simulink model "VIPLExit557StEnCtrl"  (R2018b)
settings: Solver=FixedStepDiscrete  StartTime=0.0  StopTime=10.0  FixedStep=0.01  RelTol=1e-3
undefined symbols (not defined in the file or in its folder): data, KeSMSw4SSecRwLtStLgrstOtwdInwdClosePos1_Val, KeSMSw4SSecRwLtStLgrstUpwdDnwdClosePos1_Val, KeSMSw4SSecRwLtStLgrstUpwdDnwdClosePos2_Val, KeSMSw4SSecRwLtStLgrstUpwdDnwdOpenPos1_Val, SecRwLtStBkReclnEn_Clear, SecRwLtStBkReclnEn_Set, SecRwLtStFwdBkwdEn_Clear, SecRwLtStFwdBkwdEn_Set, SecRwLtStLgrstInwdOtwdEn_Clear, SecRwLtStLgrstInwdOtwdEn_Set, SecRwLtStLgrstUpwdDnwdEn_Clear, SecRwLtStLgrstUpwdDnwdEn_Set, ThdRwLtStBkReclnEn_Clear, ThdRwLtStBkReclnEn_Set, ThdRwLtStFwdBkwdEn_Clear, ThdRwLtStFwdBkwdEn_Set, ZeroLEn_Clear, ZeroLEn_Set
libraries: simulink x1
settings Model: Creator=sn2xws  LastModifiedBy=sn2xws
settings Model: ModifiedHistory=|
  | 2024.7.2 V3.0.0 557模式流程V1.9
  | 2024.8.21 V3.0.1 增加FitstTrig参数
  | 2024.9.18 V3.0.2 三排占座应不动三排，第三阶段遗漏三排靠背动作
  | 2024.10.8 V3.0.3方向比较类型设置错误
settings DataIOCC: SaveFormat=StructureWithTime
settings OptimizationCC: DefaultParameterBehavior=Inlined  EnhancedBackFolding=on  PassReuseOutputArgsAs=Individual arguments  ZeroExternalMemoryAtStartup=off  ZeroInternalMemoryAtStartup=off  OptimizeBlockOrder=speed  DifferentSizesBufferReuse=on  OptimizationCustomize=off
settings DebuggingCC: ParameterTunabilityLossMsg=error
settings SFSimCC: MATLABDynamicMemAlloc=off
settings RTWCC: SystemTargetFile=autosar.tlc  GenCodeOnly=on  TemplateMakefile=ert_default_tmf  Description=AUTOSAR  GenerateReport=on  IncludeHyperlinkInReport=on  LaunchReport=on  GenerateTraceInfo=on  GenerateTraceReport=on  GenerateTraceReportSl=on  GenerateTraceReportSf=on  GenerateTraceReportEml=on
settings CodeAppCC: ForceParamTrailComments=on  IgnoreCustomStorageClasses=off  OperatorAnnotations=on  SimulinkDataObjDesc=on  SFDataObjDesc=on  InsertBlockDesc=on
settings STFCustomTargetCC: TargetLangStandard=C99 (ISO)  MultiwordLength=256  ParMdlRefBuildCompliant=on  CompOptLevelCompliant=on  IncludeMdlTerminateFcn=off  CombineOutputUpdateFcns=on  SuppressErrorStatus=on  ERTCustomFileBanners=on  SupportNonFinite=off  SupportComplex=off  SupportContinuousTime=off  SupportNonInlinedSFcns=off  RemoveResetFunc=on  MATLABClassNameForMDSCustomization=Simulink.SoftwareTarget.ERTCustomization  AutosarCompliant=on  UseToolchainInfoCompliant=on  LookupTableObjectStructAxisOrder=2,1,3,4,...  LUTObjectStructOrderEvenSpacing=Size,Table,Breakpoints  SystemTargetFile=autosar.tlc
settings ERTTargetCC: TargetLangStandard=C99 (ISO)  ConcurrentExecutionCompliant=off  IncludeMdlTerminateFcn=off  SuppressErrorStatus=on  SupportNonFinite=off  SupportComplex=off  ModelStepFunctionPrototypeControlCompliant=off  CPPClassGenCompliant=off  AutosarCompliant=on  LookupTableObjectStructAxisOrder=2,1,3,4,...  LUTObjectStructOrderEvenSpacing=Size,Table,Breakpoints  InlinedParameterPlacement=NonHierarchical  ERTCustomFileTemplate=example_file_process.tlc  ERTFilePackagingFormat=Compact

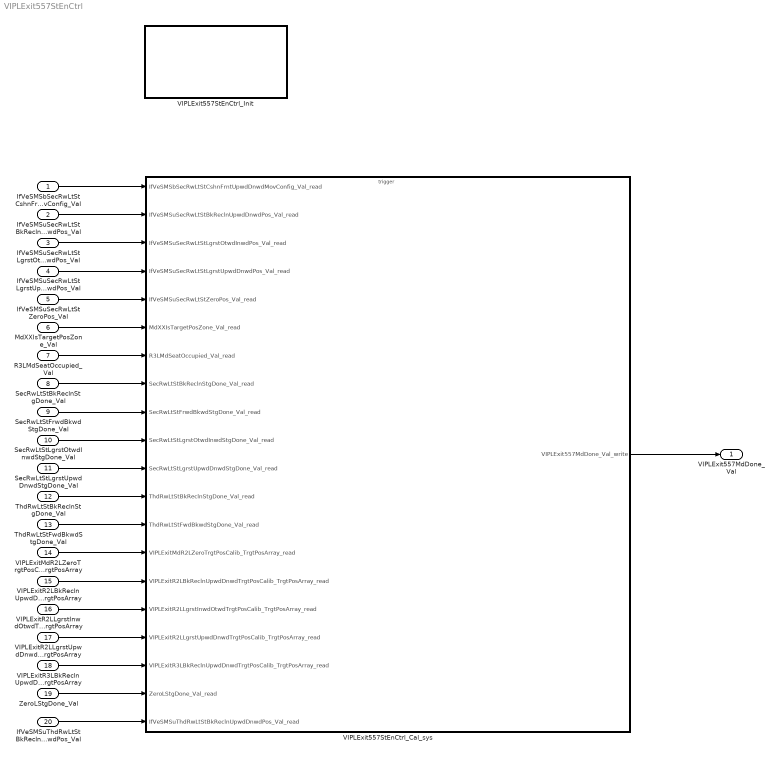
== system VIPLExit557StEnCtrl ==
  IfVeSMSbSecRwLtStCshnFrntUpwdDnwdMovConfig_Val : Inport  OutDataTypeStr=boolean  PortDimensions=1
  IfVeSMSuSecRwLtStBkReclnUpwdDnwdPos_Val : Inport  Port=2  OutDataTypeStr=uint16  PortDimensions=1
  IfVeSMSuSecRwLtStLgrstOtwdInwdPos_Val : Inport  Port=3  OutDataTypeStr=uint16  PortDimensions=1
  IfVeSMSuSecRwLtStLgrstUpwdDnwdPos_Val : Inport  Port=4  OutDataTypeStr=uint16  PortDimensions=1
  IfVeSMSuSecRwLtStZeroPos_Val : Inport  Port=5  OutDataTypeStr=uint16  PortDimensions=1
  MdXXIsTargetPosZone_Val : Inport  Port=6  OutDataTypeStr=uint32  PortDimensions=1
  R3LMdSeatOccupied_Val : Inport  Port=7  OutDataTypeStr=boolean  PortDimensions=1
  SecRwLtStBkReclnStgDone_Val : Inport  Port=8  OutDataTypeStr=boolean  PortDimensions=1
  SecRwLtStFrwdBkwdStgDone_Val : Inport  Port=9  OutDataTypeStr=boolean  PortDimensions=1
  SecRwLtStLgrstOtwdInwdStgDone_Val : Inport  Port=10  OutDataTypeStr=boolean  PortDimensions=1
  SecRwLtStLgrstUpwdDnwdStgDone_Val : Inport  Port=11  OutDataTypeStr=boolean  PortDimensions=1
  ThdRwLtStBkReclnStgDone_Val : Inport  Port=12  OutDataTypeStr=boolean  PortDimensions=1
  ThdRwLtStFwdBkwdStgDone_Val : Inport  Port=13  OutDataTypeStr=boolean  PortDimensions=1
  VIPLExitMdR2LZeroTrgtPosCalib_TrgtPosArray : Inport  Description=|  Port=14  OutDataTypeStr=uint16  PortDimensions=3
      | 0:Pos
      | 1:Max
      | 2:Min
  VIPLExitR2LBkReclnUpwdDnwdTrgtPosCalib_TrgtPosArray : Inport  Description=|  Port=15  OutDataTypeStr=uint16  PortDimensions=3
      | 0:Pos
      | 1:Max
      | 2:Min
  VIPLExitR2LLgrstInwdOtwdTrgtPosCalib_TrgtPosArray : Inport  Description=|  Port=16  OutDataTypeStr=uint16  PortDimensions=3
      | 0:Pos
      | 1:Max
      | 2:Min
  VIPLExitR2LLgrstUpwdDnwdTrgtPosCalib_TrgtPosArray : Inport  Description=|  Port=17  OutDataTypeStr=uint16  PortDimensions=3
      | 0:Pos
      | 1:Max
      | 2:Min
  VIPLExitR3LBkReclnUpwdDnwdTrgtPosCalib_TrgtPosArray : Inport  Description=|  Port=18  OutDataTypeStr=uint16  PortDimensions=3
      | 0:Pos
      | 1:Max
      | 2:Min
  ZeroLStgDone_Val : Inport  Port=19  OutDataTypeStr=boolean  PortDimensions=1
  IfVeSMSuThdRwLtStBkReclnUpwdDnwdPos_Val : Inport  Port=20  OutDataTypeStr=uint16  PortDimensions=1
  VIPLExit557StEnCtrl_Cal_sys : Subsystem
  VIPLExit557StEnCtrl_Init : Subsystem
  VIPLExit557MdDone_Val : Outport  OutDataTypeStr=uint8  PortDimensions=1
  wires:
  IfVeSMSbSecRwLtStCshnFrntUpwdDnwdMovConfig_Val/1 -> VIPLExit557StEnCtrl_Cal_sys/1(IfVeSMSbSecRwLtStCshnFrntUpwdDnwdMovConfig_Val_read)
  IfVeSMSuSecRwLtStBkReclnUpwdDnwdPos_Val/1 -> VIPLExit557StEnCtrl_Cal_sys/2(IfVeSMSuSecRwLtStBkReclnUpwdDnwdPos_Val_read)
  IfVeSMSuSecRwLtStLgrstOtwdInwdPos_Val/1 -> VIPLExit557StEnCtrl_Cal_sys/3(IfVeSMSuSecRwLtStLgrstOtwdInwdPos_Val_read)
  IfVeSMSuSecRwLtStLgrstUpwdDnwdPos_Val/1 -> VIPLExit557StEnCtrl_Cal_sys/4(IfVeSMSuSecRwLtStLgrstUpwdDnwdPos_Val_read)
  IfVeSMSuSecRwLtStZeroPos_Val/1 -> VIPLExit557StEnCtrl_Cal_sys/5(IfVeSMSuSecRwLtStZeroPos_Val_read)
  MdXXIsTargetPosZone_Val/1 -> VIPLExit557StEnCtrl_Cal_sys/6(MdXXIsTargetPosZone_Val_read)
  R3LMdSeatOccupied_Val/1 -> VIPLExit557StEnCtrl_Cal_sys/7(R3LMdSeatOccupied_Val_read)
  SecRwLtStBkReclnStgDone_Val/1 -> VIPLExit557StEnCtrl_Cal_sys/8(SecRwLtStBkReclnStgDone_Val_read)
  SecRwLtStFrwdBkwdStgDone_Val/1 -> VIPLExit557StEnCtrl_Cal_sys/9(SecRwLtStFrwdBkwdStgDone_Val_read)
  SecRwLtStLgrstOtwdInwdStgDone_Val/1 -> VIPLExit557StEnCtrl_Cal_sys/10(SecRwLtStLgrstOtwdInwdStgDone_Val_read)
  SecRwLtStLgrstUpwdDnwdStgDone_Val/1 -> VIPLExit557StEnCtrl_Cal_sys/11(SecRwLtStLgrstUpwdDnwdStgDone_Val_read)
  ThdRwLtStBkReclnStgDone_Val/1 -> VIPLExit557StEnCtrl_Cal_sys/12(ThdRwLtStBkReclnStgDone_Val_read)
  ThdRwLtStFwdBkwdStgDone_Val/1 -> VIPLExit557StEnCtrl_Cal_sys/13(ThdRwLtStFwdBkwdStgDone_Val_read)
  VIPLExitMdR2LZeroTrgtPosCalib_TrgtPosArray/1 -> VIPLExit557StEnCtrl_Cal_sys/14(VIPLExitMdR2LZeroTrgtPosCalib_TrgtPosArray_read)
  VIPLExitR2LBkReclnUpwdDnwdTrgtPosCalib_TrgtPosArray/1 -> VIPLExit557StEnCtrl_Cal_sys/15(VIPLExitR2LBkReclnUpwdDnwdTrgtPosCalib_TrgtPosArray_read)
  VIPLExitR2LLgrstInwdOtwdTrgtPosCalib_TrgtPosArray/1 -> VIPLExit557StEnCtrl_Cal_sys/16(VIPLExitR2LLgrstInwdOtwdTrgtPosCalib_TrgtPosArray_read)
  VIPLExitR2LLgrstUpwdDnwdTrgtPosCalib_TrgtPosArray/1 -> VIPLExit557StEnCtrl_Cal_sys/17(VIPLExitR2LLgrstUpwdDnwdTrgtPosCalib_TrgtPosArray_read)
  VIPLExitR3LBkReclnUpwdDnwdTrgtPosCalib_TrgtPosArray/1 -> VIPLExit557StEnCtrl_Cal_sys/18(VIPLExitR3LBkReclnUpwdDnwdTrgtPosCalib_TrgtPosArray_read)
  ZeroLStgDone_Val/1 -> VIPLExit557StEnCtrl_Cal_sys/19(ZeroLStgDone_Val_read)
  VIPLExit557StEnCtrl_Cal_sys/1(VIPLExit557MdDone_Val_write) -> VIPLExit557MdDone_Val/1
  IfVeSMSuThdRwLtStBkReclnUpwdDnwdPos_Val/1 -> VIPLExit557StEnCtrl_Cal_sys/20(IfVeSMSuThdRwLtStBkReclnUpwdDnwdPos_Val_read)

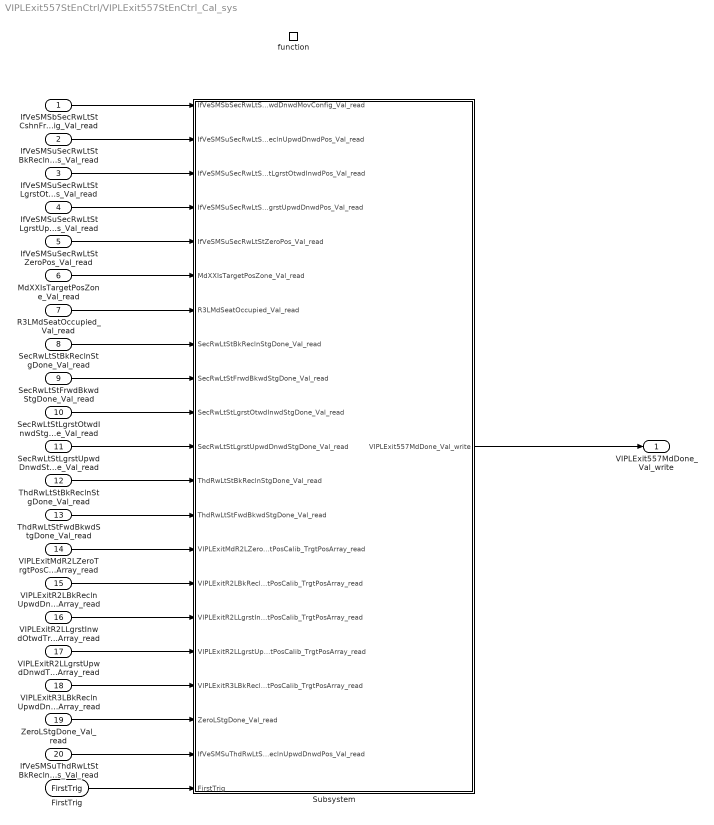
== system VIPLExit557StEnCtrl/VIPLExit557StEnCtrl_Cal_sys ==
  IfVeSMSbSecRwLtStCshnFrntUpwdDnwdMovConfig_Val_read : Inport
  IfVeSMSuSecRwLtStBkReclnUpwdDnwdPos_Val_read : Inport  Port=2
  IfVeSMSuSecRwLtStLgrstOtwdInwdPos_Val_read : Inport  Port=3
  IfVeSMSuSecRwLtStLgrstUpwdDnwdPos_Val_read : Inport  Port=4
  IfVeSMSuSecRwLtStZeroPos_Val_read : Inport  Port=5
  MdXXIsTargetPosZone_Val_read : Inport  Port=6
  R3LMdSeatOccupied_Val_read : Inport  Port=7
  SecRwLtStBkReclnStgDone_Val_read : Inport  Port=8
  SecRwLtStFrwdBkwdStgDone_Val_read : Inport  Port=9
  SecRwLtStLgrstOtwdInwdStgDone_Val_read : Inport  Port=10
  SecRwLtStLgrstUpwdDnwdStgDone_Val_read : Inport  Port=11
  ThdRwLtStBkReclnStgDone_Val_read : Inport  Port=12
  ThdRwLtStFwdBkwdStgDone_Val_read : Inport  Port=13
  VIPLExitMdR2LZeroTrgtPosCalib_TrgtPosArray_read : Inport  Port=14
  VIPLExitR2LBkReclnUpwdDnwdTrgtPosCalib_TrgtPosArray_read : Inport  Port=15
  VIPLExitR2LLgrstInwdOtwdTrgtPosCalib_TrgtPosArray_read : Inport  Port=16
  VIPLExitR2LLgrstUpwdDnwdTrgtPosCalib_TrgtPosArray_read : Inport  Port=17
  VIPLExitR3LBkReclnUpwdDnwdTrgtPosCalib_TrgtPosArray_read : Inport  Port=18
  ZeroLStgDone_Val_read : Inport  Port=19
  IfVeSMSuThdRwLtStBkReclnUpwdDnwdPos_Val_read : Inport  Port=20
  function : TriggerPort  TriggerType=function-call  IsSimulinkFunction=on  FunctionName=VIPLExit557StEnCtrl_Cal  VariantControl=(inherit)
  Subsystem : Subsystem
  FirstTrig : ArgIn  OutDataTypeStr=boolean  ArgumentName=FirstTrig
  VIPLExit557MdDone_Val_write : Outport
      settings: EnsureOutportIsVirtual=on
  wires:
  IfVeSMSbSecRwLtStCshnFrntUpwdDnwdMovConfig_Val_read/1 -> Subsystem/1(IfVeSMSbSecRwLtStCshnFrntUpwdDnwdMovConfig_Val_read)
  IfVeSMSuSecRwLtStBkReclnUpwdDnwdPos_Val_read/1 -> Subsystem/2(IfVeSMSuSecRwLtStBkReclnUpwdDnwdPos_Val_read)
  IfVeSMSuSecRwLtStLgrstOtwdInwdPos_Val_read/1 -> Subsystem/3(IfVeSMSuSecRwLtStLgrstOtwdInwdPos_Val_read)
  IfVeSMSuSecRwLtStLgrstUpwdDnwdPos_Val_read/1 -> Subsystem/4(IfVeSMSuSecRwLtStLgrstUpwdDnwdPos_Val_read)
  IfVeSMSuSecRwLtStZeroPos_Val_read/1 -> Subsystem/5(IfVeSMSuSecRwLtStZeroPos_Val_read)
  MdXXIsTargetPosZone_Val_read/1 -> Subsystem/6(MdXXIsTargetPosZone_Val_read)
  R3LMdSeatOccupied_Val_read/1 -> Subsystem/7(R3LMdSeatOccupied_Val_read)
  SecRwLtStBkReclnStgDone_Val_read/1 -> Subsystem/8(SecRwLtStBkReclnStgDone_Val_read)
  SecRwLtStFrwdBkwdStgDone_Val_read/1 -> Subsystem/9(SecRwLtStFrwdBkwdStgDone_Val_read)
  SecRwLtStLgrstOtwdInwdStgDone_Val_read/1 -> Subsystem/10(SecRwLtStLgrstOtwdInwdStgDone_Val_read)
  SecRwLtStLgrstUpwdDnwdStgDone_Val_read/1 -> Subsystem/11(SecRwLtStLgrstUpwdDnwdStgDone_Val_read)
  ThdRwLtStBkReclnStgDone_Val_read/1 -> Subsystem/12(ThdRwLtStBkReclnStgDone_Val_read)
  ThdRwLtStFwdBkwdStgDone_Val_read/1 -> Subsystem/13(ThdRwLtStFwdBkwdStgDone_Val_read)
  VIPLExitMdR2LZeroTrgtPosCalib_TrgtPosArray_read/1 -> Subsystem/14(VIPLExitMdR2LZeroTrgtPosCalib_TrgtPosArray_read)
  VIPLExitR2LBkReclnUpwdDnwdTrgtPosCalib_TrgtPosArray_read/1 -> Subsystem/15(VIPLExitR2LBkReclnUpwdDnwdTrgtPosCalib_TrgtPosArray_read)
  VIPLExitR2LLgrstInwdOtwdTrgtPosCalib_TrgtPosArray_read/1 -> Subsystem/16(VIPLExitR2LLgrstInwdOtwdTrgtPosCalib_TrgtPosArray_read)
  VIPLExitR2LLgrstUpwdDnwdTrgtPosCalib_TrgtPosArray_read/1 -> Subsystem/17(VIPLExitR2LLgrstUpwdDnwdTrgtPosCalib_TrgtPosArray_read)
  VIPLExitR3LBkReclnUpwdDnwdTrgtPosCalib_TrgtPosArray_read/1 -> Subsystem/18(VIPLExitR3LBkReclnUpwdDnwdTrgtPosCalib_TrgtPosArray_read)
  ZeroLStgDone_Val_read/1 -> Subsystem/19(ZeroLStgDone_Val_read)
  Subsystem/1(VIPLExit557MdDone_Val_write) -> VIPLExit557MdDone_Val_write/1
  IfVeSMSuThdRwLtStBkReclnUpwdDnwdPos_Val_read/1 -> Subsystem/20(IfVeSMSuThdRwLtStBkReclnUpwdDnwdPos_Val_read)
  FirstTrig/1 -> Subsystem/21(FirstTrig)

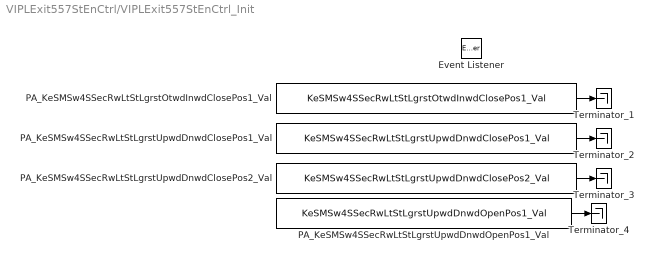
== system VIPLExit557StEnCtrl/VIPLExit557StEnCtrl_Init ==
  Event Listener : EventListener  EventName=reset
  PA_KeSMSw4SSecRwLtStLgrstOtwdInwdClosePos1_Val : Constant  Value=KeSMSw4SSecRwLtStLgrstOtwdInwdClosePos1_Val
  PA_KeSMSw4SSecRwLtStLgrstUpwdDnwdClosePos1_Val : Constant  Value=KeSMSw4SSecRwLtStLgrstUpwdDnwdClosePos1_Val
  PA_KeSMSw4SSecRwLtStLgrstUpwdDnwdClosePos2_Val : Constant  Value=KeSMSw4SSecRwLtStLgrstUpwdDnwdClosePos2_Val
  PA_KeSMSw4SSecRwLtStLgrstUpwdDnwdOpenPos1_Val : Constant  Value=KeSMSw4SSecRwLtStLgrstUpwdDnwdOpenPos1_Val
  Terminator_{1..4} (4 alike) : Terminator
  wires:
  PA_KeSMSw4SSecRwLtStLgrstOtwdInwdClosePos1_Val/1 -> Terminator_1/1
  PA_KeSMSw4SSecRwLtStLgrstUpwdDnwdClosePos1_Val/1 -> Terminator_2/1
  PA_KeSMSw4SSecRwLtStLgrstUpwdDnwdClosePos2_Val/1 -> Terminator_3/1
  PA_KeSMSw4SSecRwLtStLgrstUpwdDnwdOpenPos1_Val/1 -> Terminator_4/1

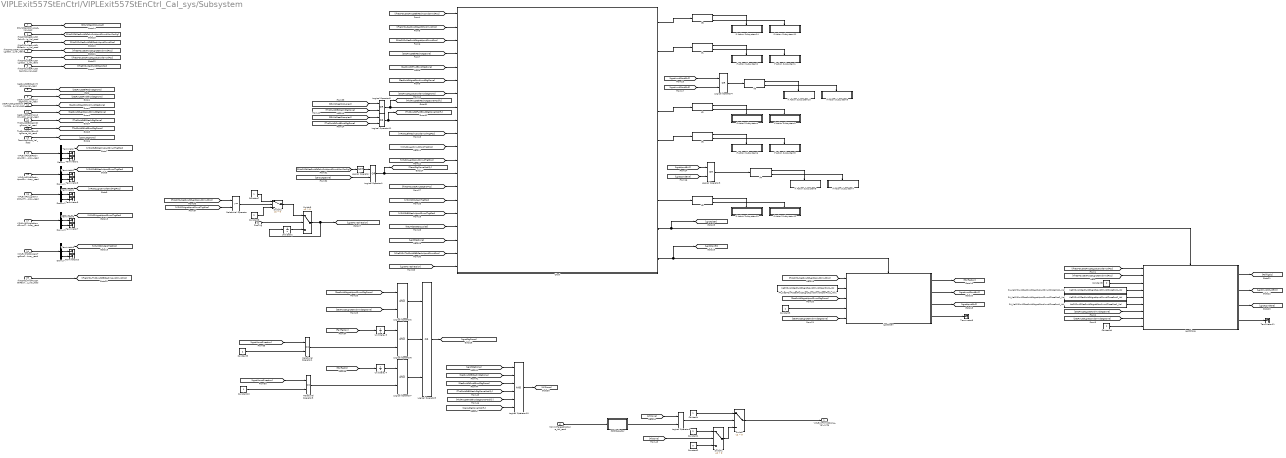
== system VIPLExit557StEnCtrl/VIPLExit557StEnCtrl_Cal_sys/Subsystem ==
  IfVeSMSbSecRwLtStCshnFrntUpwdDnwdMovConfig_Val_read : Inport
  IfVeSMSuSecRwLtStBkReclnUpwdDnwdPos_Val_read : Inport  Port=2
  IfVeSMSuSecRwLtStLgrstOtwdInwdPos_Val_read : Inport  Port=3
  IfVeSMSuSecRwLtStLgrstUpwdDnwdPos_Val_read : Inport  Port=4
  IfVeSMSuSecRwLtStZeroPos_Val_read : Inport  Port=5
  MdXXIsTargetPosZone_Val_read : Inport  Port=6
  R3LMdSeatOccupied_Val_read : Inport  Port=7
  SecRwLtStBkReclnStgDone_Val_read : Inport  Port=8
  SecRwLtStFrwdBkwdStgDone_Val_read : Inport  Port=9
  SecRwLtStLgrstOtwdInwdStgDone_Val_read : Inport  Port=10
  SecRwLtStLgrstUpwdDnwdStgDone_Val_read : Inport  Port=11
  ThdRwLtStBkReclnStgDone_Val_read : Inport  Port=12
  ThdRwLtStFwdBkwdStgDone_Val_read : Inport  Port=13
  VIPLExitMdR2LZeroTrgtPosCalib_TrgtPosArray_read : Inport  Port=14
  VIPLExitR2LBkReclnUpwdDnwdTrgtPosCalib_TrgtPosArray_read : Inport  Port=15
  VIPLExitR2LLgrstInwdOtwdTrgtPosCalib_TrgtPosArray_read : Inport  Port=16
  VIPLExitR2LLgrstUpwdDnwdTrgtPosCalib_TrgtPosArray_read : Inport  Port=17
  VIPLExitR3LBkReclnUpwdDnwdTrgtPosCalib_TrgtPosArray_read : Inport  Port=18
  ZeroLStgDone_Val_read : Inport  Port=19
  IfVeSMSuThdRwLtStBkReclnUpwdDnwdPos_Val_read : Inport  Port=20
  FirstTrig : Inport  Port=21
  32BitSelector : Subsystem  mask(32 Bit Selector){BitNum=26}
      mask prompts: BitNum "Select Bit Number"
      mask help: Allows selection of a particular bit (0-31) out of a packed word up to 32 bits long. Output will be true if the bit number selected via the mask parameter is equal to one.
      mask TypeOptions BitNum: 0 | 1 | 2 | 3 | 4 | 5 | 6 | 7 | 8 | 9 | 10 | 11 | 12 | 13 | 14 | 15 | 16 | 17 | 18 | 19 | 20 | 21 | 22 | 23 | 24 | 25 | 26 | 27 | 28 | 29 | 30 | 31
      mask Display:
      | text(0.5, 0.8,'BIT','horizontalAlignment','center')
      | text(0.5, 0.5,'SELECTOR','horizontalAlignment','center')
      | text(0.5, 0.2,['-- Bit ',char(get_param(gcb,'BitNum')),' --'],'horizontalAlignment','center')
  Chart : Stateflow chart  TreatAsAtomicUnit=on
  Constant : Constant  OutDataTypeStr=uint8
  Constant1 : Constant  Value=2  OutDataTypeStr=uint8
  Constant10 : Constant  OutDataTypeStr=uint8
  Constant2 : Constant  Value=0  OutDataTypeStr=uint8
  Constant3 : Constant  OutDataTypeStr=boolean
  Constant4 : Constant  OutDataTypeStr=boolean
  Constant5 : Constant  Value=0  OutDataTypeStr=uint16
  Constant7 : Constant  OutDataTypeStr=uint8
  Constant8 : Constant  Value=2  OutDataTypeStr=uint8
  Constant9 : Constant  Value=2  OutDataTypeStr=uint8
  Demux{,1..4} (5 alike) : Demux  Outputs=3
  If Action Subsystem1 : Subsystem  TreatAsAtomicUnit=on
  If Action Subsystem10 : Subsystem  TreatAsAtomicUnit=on
  If Action Subsystem11 : Subsystem  TreatAsAtomicUnit=on
  If Action Subsystem12 : Subsystem  TreatAsAtomicUnit=on
  If Action Subsystem13 : Subsystem  TreatAsAtomicUnit=on
  If Action Subsystem14 : Subsystem  TreatAsAtomicUnit=on
  If Action Subsystem2 : Subsystem  TreatAsAtomicUnit=on
  If Action Subsystem3 : Subsystem  TreatAsAtomicUnit=on
  If Action Subsystem4 : Subsystem  TreatAsAtomicUnit=on
  If Action Subsystem5 : Subsystem  TreatAsAtomicUnit=on
  If Action Subsystem6 : Subsystem  TreatAsAtomicUnit=on
  If Action Subsystem7 : Subsystem  TreatAsAtomicUnit=on
  If Action Subsystem8 : Subsystem  TreatAsAtomicUnit=on
  If Action Subsystem9 : Subsystem  TreatAsAtomicUnit=on
  If{1..6,8} (7 alike) : If  IfExpression=u1
  LgrstClose : Subsystem
  LgrstOpen : Subsystem
  Logical Operator : Logic  Operator=NOT  AllPortsSameDT=off  OutDataTypeStr=boolean
  Logical Operator{1,3..4,8,11} (5 alike) : Logic  Operator=OR  AllPortsSameDT=off  OutDataTypeStr=boolean
  Logical Operator10 : Logic  Inputs=6  AllPortsSameDT=off  OutDataTypeStr=boolean
  Logical Operator{2,6..7,9} (4 alike) : Logic  AllPortsSameDT=off  OutDataTypeStr=boolean
  Logical Operator5 : Logic  Operator=OR  Inputs=3  AllPortsSameDT=off  OutDataTypeStr=boolean
  PA_KeSMSw4SSecRwLtStLgrstOtwdInwdClosePos1_Val : Constant  Value=KeSMSw4SSecRwLtStLgrstOtwdInwdClosePos1_Val
  PA_KeSMSw4SSecRwLtStLgrstUpwdDnwdClosePos1_Val : Constant  Value=KeSMSw4SSecRwLtStLgrstUpwdDnwdClosePos1_Val
  PA_KeSMSw4SSecRwLtStLgrstUpwdDnwdClosePos2_Val : Constant  Value=KeSMSw4SSecRwLtStLgrstUpwdDnwdClosePos2_Val
  PA_KeSMSw4SSecRwLtStLgrstUpwdDnwdOpenPos1_Val1 : Constant  Value=KeSMSw4SSecRwLtStLgrstUpwdDnwdOpenPos1_Val
  Relational Operator : RelationalOperator  OutDataTypeStr=boolean  RndMeth=Simplest
  Relational Operator1 : RelationalOperator  Operator===  OutDataTypeStr=boolean  RndMeth=Simplest
  Relational Operator3 : RelationalOperator  Operator===  OutDataTypeStr=boolean  RndMeth=Simplest
  Switch{,1..2,5} (4 alike) : Switch  Criteria=u2 > Threshold
  Terminator{,1..11} (12 alike) : Terminator
  Unit Delay : UnitDelay  SampleTime=-1
  Unit Delay3 : UnitDelay  SampleTime=-1
  Unit Delay4 : UnitDelay  SampleTime=-1
  VIPLExit557MdDone_Val_write : Outport
      settings: EnsureOutportIsVirtual=on
  wires:
  Switch/1 -> VIPLExit557MdDone_Val_write/1
  Constant1/1 -> Switch1/1
  Constant/1 -> Switch/1
  Constant2/1 -> Switch1/3
  32BitSelector/1(y) -> Logical Operator9/2
  Switch1/1 -> Switch/3
  MdXXIsTargetPosZone_Val_read/1 -> 32BitSelector/1(x)
  [AllDone] -> Logical Operator9/1
  [AllDone] -> Switch1/2
  Logical Operator9/1 -> Switch/2
  ZeroLStgDone_Val_read/1 -> [ZeroLStgDone]
  IfVeSMSuSecRwLtStBkReclnUpwdDnwdPos_Val_read/1 -> [IfVeSMSuSecRwLtStBkReclnUpwdDnwdPos]
  SecRwLtStLgrstUpwdDnwdStgDone_Val_read/1 -> [SecRwLtStLgrstUpwdDnwdStgDone]
  IfVeSMSuSecRwLtStLgrstUpwdDnwdPos_Val_read/1 -> [IfVeSMSuSecRwLtStLgrstUpwdDnwdPos]
  SecRwLtStFrwdBkwdStgDone_Val_read/1 -> [SecRwLtStFrwdBkwdStgDone]
  IfVeSMSuSecRwLtStLgrstOtwdInwdPos_Val_read/1 -> [IfVeSMSuSecRwLtStLgrstOtwdInwdPos]
  SecRwLtStLgrstOtwdInwdStgDone_Val_read/1 -> [SecRwLtStLgrstOtwdInwdStgDone]
  ThdRwLtStBkReclnStgDone_Val_read/1 -> [ThdRwLtStBkReclnStgDone]
  ThdRwLtStFwdBkwdStgDone_Val_read/1 -> [ThdRwLtStFwdBkwdStgDone]
  SecRwLtStBkReclnStgDone_Val_read/1 -> [SecRwLtStBkReclnStgDone]
  IfVeSMSuSecRwLtStZeroPos_Val_read/1 -> [IfVeSMSuSecRwLtStZeroPos]
  Demux4/3 -> Terminator10/1
  VIPLExitR3LBkReclnUpwdDnwdTrgtPosCalib_TrgtPosArray_read/1 -> Demux/1
  Demux4/2 -> Terminator9/1
  VIPLExitMdR2LZeroTrgtPosCalib_TrgtPosArray_read/1 -> Demux4/1
  Demux3/1 -> [VIPLR2LLgrstUpwdDnwdTrgtPos]
  Demux2/2 -> Terminator4/1
  Demux1/3 -> Terminator3/1
  Demux1/2 -> Terminator2/1
  Demux1/1 -> [VIPLR2LBkReclnUpwdDnwdTrgtPos]
  Demux/2 -> Terminator/1
  Demux3/3 -> Terminator7/1
  Demux2/1 -> [VIPLR2LLgrstInwdOtwdTrgtPos]
  Demux/3 -> Terminator1/1
  Demux4/1 -> [VIPLMdR2LZeroTrgtPos]
  VIPLExitR2LBkReclnUpwdDnwdTrgtPosCalib_TrgtPosArray_read/1 -> Demux1/1
  VIPLExitR2LLgrstInwdOtwdTrgtPosCalib_TrgtPosArray_read/1 -> Demux2/1
  Demux3/2 -> Terminator6/1
  Demux2/3 -> Terminator5/1
  Demux/1 -> [VIPLR3LBkReclnUpwdDnwdTrgtPos]
  VIPLExitR2LLgrstUpwdDnwdTrgtPosCalib_TrgtPosArray_read/1 -> Demux3/1
  R3LMdSeatOccupied_Val_read/1 -> [R3LMdSeatOccupied]
  IfVeSMSbSecRwLtStCshnFrntUpwdDnwdMovConfig_Val_read/1 -> [IfVeSMSbSecRwLtStCshnFrntUpwdDnwdMovConfig]
  [SecRwLtStLgrstOtwdInwdStgDone] -> LgrstOpen/5(LgrstInwdStgDone)
  LgrstOpen/1(Failflg) -> [FailflgOpn]
  LgrstOpen/4(FtrstEn) -> Terminator8/1
  PA_KeSMSw4SSecRwLtStLgrstUpwdDnwdOpenPos1_Val1/1 -> LgrstOpen/2(LgrstUpwdDnwdOpenPos1)
  Constant3/1 -> LgrstOpen/4(FtrstStgDone)
  LgrstOpen/2(LgrstInwdOtwdEn) -> [LgrstInwdOtwdEn2]
  LgrstOpen/3(LgrstUpwdDnwdEn) -> [LgrstUpwdEn2]
  [SecRwLtStLgrstUpwdDnwdStgDone] -> LgrstOpen/3(LgrstUpwdStgDone)
  [IfVeSMSuSecRwLtStLgrstUpwdDnwdPos] -> LgrstOpen/1(LgrstUpwdDnwdPos)
  PA_KeSMSw4SSecRwLtStLgrstOtwdInwdClosePos1_Val/1 -> LgrstClose/6(LgrstInwdOtWdPos1)
  PA_KeSMSw4SSecRwLtStLgrstUpwdDnwdClosePos1_Val/1 -> LgrstClose/4(LgrstUpwdDnwdClosePos1)
  PA_KeSMSw4SSecRwLtStLgrstUpwdDnwdClosePos2_Val/1 -> LgrstClose/5(LgrstUpwdDnwdClosePos2)
  Constant4/1 -> LgrstClose/9(FtrstStgDone)
  Constant5/1 -> LgrstClose/3(FtupwdDnwdPos)
  [IfVeSMSuSecRwLtStLgrstOtwdInwdPos] -> LgrstClose/2(LgrstInwdOtwdPos)
  [IfVeSMSuSecRwLtStLgrstUpwdDnwdPos] -> LgrstClose/1(LgrstUpwdDnwdPos)
  [SecRwLtStLgrstUpwdDnwdStgDone] -> LgrstClose/8(LgrstUpwdStgDone)
  [SecRwLtStLgrstOtwdInwdStgDone] -> LgrstClose/7(LgrstInwdStgDone)
  LgrstClose/1(Failflg) -> [FailflgCls]
  LgrstClose/2(LgrstInwdOtwdEn) -> [LgrstInwdOtwdEn3]
  LgrstClose/3(LgrstUpwdDnwdEn) -> [LgrstUpwdEn3]
  LgrstClose/4(FtrstEn) -> Terminator11/1
  [IfVeSMSuSecRwLtStLgrstOtwdInwdPos] -> Chart/2(IfVeSMSuSecRwLtStLgrstOtwdInwdPos)
  [SecRwLtStLgrstOtwdInwdStgDone] -> Chart/6(SecRwLtStLgrstOtwdInwdStgDone)
  [VIPLR2LBkReclnUpwdDnwdTrgtPos] -> Chart/10(VIPLR2LBkReclnUpwdDnwdTrgtPos)
  If6/2 -> If Action Subsystem12/Action
  Chart/7(ZeroLEn) -> If6/1
  Logical Operator1/1 -> [ZeroLStgDoneModify], Chart/13(ZeroLStgDone)
  Logical Operator3/1 -> If4/1
  If4/1 -> If Action Subsystem8/Action
  Chart/4(ThdRwLtStBkReclnEn) -> If2/1
  If4/2 -> If Action Subsystem7/Action
  Chart/2(SecRwLtStFrwdBkwdEn) -> If1/1
  [VIPLR2LLgrstUpwdDnwdTrgtPos] -> Chart/12(VIPLR2LLgrstUpwdDnwdTrgtPos)
  [IfVeSMSuSecRwLtStZeroPos] -> Chart/14(IfVeSMSuSecRwLtStZeroPos)
  [IfVeSMSuSecRwLtStBkReclnUpwdDnwdPos] -> Chart/1(IfVeSMSuSecRwLtStBkReclnUpwdDnwdPos)
  [SecRwLtStLgrstUpwdDnwdStgDone] -> Chart/7(SecRwLtStLgrstUpwdDnwdStgDone)
  [SecRwLtStFrwdBkwdStgDone] -> Chart/5(SecRwLtStFrwdBkwdStgDone)
  If3/1 -> If Action Subsystem6/Action
  If2/1 -> If Action Subsystem4/Action
  If8/1 -> If Action Subsystem14/Action
  If2/2 -> If Action Subsystem3/Action
  If1/2 -> If Action Subsystem1/Action
  Logical Operator4/1 -> If5/1
  If1/1 -> If Action Subsystem2/Action
  Chart/5(ThdRwLtStFwdBkwdEn) -> If3/1
  If8/2 -> If Action Subsystem11/Action
  [LgrstUpwdEn2] -> Logical Operator3/1
  [VIPLR2LLgrstInwdOtwdTrgtPos] -> Chart/11(VIPLR2LLgrstInwdOtwdTrgtPos)
  [IfVeSMSuSecRwLtStLgrstUpwdDnwdPos] -> Chart/3(IfVeSMSuSecRwLtStLgrstUpwdDnwdPos)
  [SecRwLtStBkReclnStgDone] -> Chart/4(SecRwLtStBkReclnStgDone)
  If5/2 -> If Action Subsystem9/Action
  Chart/1(SecRwLtStBkReclnEn) -> If8/1
  If6/1 -> If Action Subsystem13/Action
  [LgrstInwdOtwdEn2] -> Logical Operator4/1
  If5/1 -> If Action Subsystem10/Action
  If3/2 -> If Action Subsystem5/Action
  [VIPLMdR2LZeroTrgtPos] -> Chart/15(VIPLMdR2LZeroTrgtPos)
  [LgrstUpwdEn3] -> Logical Operator3/2
  [LgrstInwdOtwdEn3] -> Logical Operator4/2
  [VIPLR3LBkReclnUpwdDnwdTrgtPos] -> Chart/16(VIPLR3LBkReclnUpwdDnwdTrgtPos)
  [R3LMdSeatOccupied] -> Chart/17(R3LMdSeatOccupied)
  [LgrstStgDone] -> Chart/18(LgrstStgDone)
  [IfVeSMSuThdRwLtStBkReclnUpwdDnwdPos] -> Chart/19(IfVeSMSuThdRwLtStBkReclnUpwdDnwdPos)
  [IfVeSMSbSecRwLtStCshnFrntUpwdDnwdMovConfig] -> Logical Operator/1
  Logical Operator/1 -> Logical Operator1/1
  [ZeroLStgDone] -> Logical Operator1/2
  [SecRwLtStLgrstUpwdDnwdStgDone] -> Logical Operator2/1
  [SecRwLtStLgrstOtwdInwdStgDone] -> Logical Operator2/2
  Logical Operator2/1 -> Logical Operator5/1
  [FailflgOpn] -> Unit Delay3/1
  Logical Operator6/1 -> Logical Operator5/2
  [FailflgCls] -> Unit Delay4/1
  Logical Operator5/1 -> [LgrstStgDone]
  [IfVeSMSuSecRwLtStLgrstUpwdDnwdPos] -> Relational Operator/1
  [VIPLR2LLgrstUpwdDnwdTrgtPos] -> Relational Operator/2
  Relational Operator/1 -> Switch2/2
  Constant7/1 -> Switch2/1
  Constant8/1 -> Switch2/3
  [LgrstMoveDirection] -> Chart/20(LgrstMoveDirection)
  Logical Operator7/1 -> Logical Operator5/3
  Chart/9(LgrstOpnEn) -> [LgrstOpnEn], LgrstOpen/Enable
  Chart/8(LgrstClsEn) -> [LgrstClsEn], LgrstClose/Enable
  IfVeSMSuThdRwLtStBkReclnUpwdDnwdPos_Val_read/1 -> [IfVeSMSuThdRwLtStBkReclnUpwdDnwdPos]
  [LgrstStgDone] -> Logical Operator10/1
  Logical Operator10/1 -> [AllDone]
  [SecRwLtStBkReclnStgDone] -> Logical Operator10/2
  [SecRwLtStFrwdBkwdStgDone] -> Logical Operator10/3
  [ThdRwLtStBkReclnStgDoneModify] -> Logical Operator10/4
  [ThdRwLtStFwdBkwdStgDoneModify] -> Logical Operator10/5
  [ZeroLStgDoneModify] -> Logical Operator10/6
  Unit Delay3/1 -> Logical Operator6/1
  Unit Delay4/1 -> Logical Operator7/1
  FirstTrig/1 -> Switch5/2
  Switch2/1 -> Switch5/1
  Unit Delay/1 -> Switch5/3
  Switch5/1 -> Unit Delay/1, [LgrstMoveDirection]
  Relational Operator1/1 -> Logical Operator6/2
  Constant9/1 -> Relational Operator1/2
  [LgrstMoveDirection] -> Relational Operator1/1
  [LgrstMoveDirection] -> Relational Operator3/1
  Constant10/1 -> Relational Operator3/2
  Relational Operator3/1 -> Logical Operator7/2
  [R3LMdSeatOccupied] -> Logical Operator8/1
  [ThdRwLtStBkReclnStgDone] -> Logical Operator8/2
  [R3LMdSeatOccupied] -> Logical Operator11/1
  [ThdRwLtStFwdBkwdStgDone] -> Logical Operator11/2
  Logical Operator8/1 -> [ThdRwLtStBkReclnStgDoneModify], Chart/8(ThdRwLtStBkReclnStgDone)
  Logical Operator11/1 -> [ThdRwLtStFwdBkwdStgDoneModify], Chart/9(ThdRwLtStFwdBkwdStgDone)

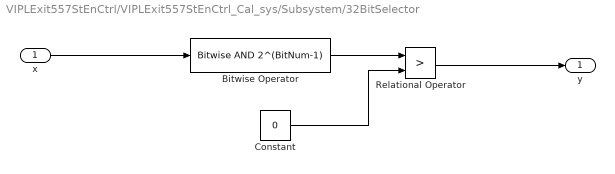
== system VIPLExit557StEnCtrl/VIPLExit557StEnCtrl_Cal_sys/Subsystem/32BitSelector ==
  x : Inport
  Bitwise Operator : simulink/Logic and Bit Operations/Bitwise Operator  logicop=AND  UseBitMask=on  BitMask=2^(BitNum-1)  BitMaskRealWorld=Stored Integer
  Constant : Constant  Value=0  OutDataTypeStr=uint32
  Relational Operator : RelationalOperator  Operator=>  OutDataTypeStr=boolean  RndMeth=Simplest
  y : Outport
  wires:
  Relational Operator/1 -> y/1
  Constant/1 -> Relational Operator/2
  x/1 -> Bitwise Operator/1
  Bitwise Operator/1 -> Relational Operator/1

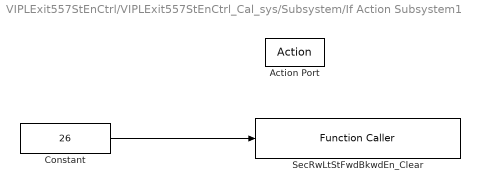
== system VIPLExit557StEnCtrl/VIPLExit557StEnCtrl_Cal_sys/Subsystem/If Action Subsystem1 ==
  Action Port : ActionPort  ActionType=else
  Constant : Constant  Value=26  OutDataTypeStr=uint8
  SecRwLtStFwdBkwdEn_Clear : FunctionCaller  FunctionPrototype=SecRwLtStFwdBkwdEn_Clear(data)  InputArgumentSpecifications=uint8(1)
  wires:
  Constant/1 -> SecRwLtStFwdBkwdEn_Clear/1

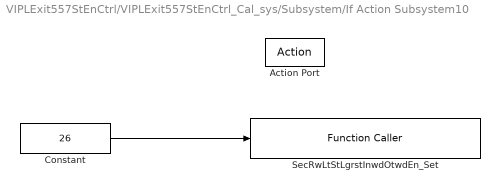
== system VIPLExit557StEnCtrl/VIPLExit557StEnCtrl_Cal_sys/Subsystem/If Action Subsystem10 ==
  Action Port : ActionPort  ActionType=then
  Constant : Constant  Value=26  OutDataTypeStr=uint8
  SecRwLtStLgrstInwdOtwdEn_Set : FunctionCaller  FunctionPrototype=SecRwLtStLgrstInwdOtwdEn_Set(data)  InputArgumentSpecifications=uint8(1)
  wires:
  Constant/1 -> SecRwLtStLgrstInwdOtwdEn_Set/1

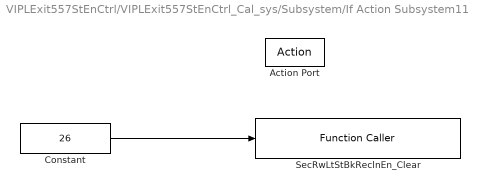
== system VIPLExit557StEnCtrl/VIPLExit557StEnCtrl_Cal_sys/Subsystem/If Action Subsystem11 ==
  Action Port : ActionPort  ActionType=else
  Constant : Constant  Value=26  OutDataTypeStr=uint8
  SecRwLtStBkReclnEn_Clear : FunctionCaller  FunctionPrototype=SecRwLtStBkReclnEn_Clear(data)  InputArgumentSpecifications=uint8(1)
  wires:
  Constant/1 -> SecRwLtStBkReclnEn_Clear/1

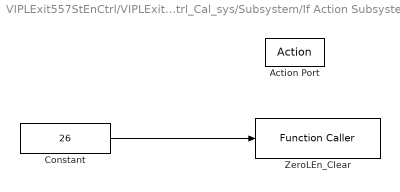
== system VIPLExit557StEnCtrl/VIPLExit557StEnCtrl_Cal_sys/Subsystem/If Action Subsystem12 ==
  Action Port : ActionPort  ActionType=else
  Constant : Constant  Value=26  OutDataTypeStr=uint8
  ZeroLEn_Clear : FunctionCaller  FunctionPrototype=ZeroLEn_Clear(data)  InputArgumentSpecifications=uint8(1)
  wires:
  Constant/1 -> ZeroLEn_Clear/1

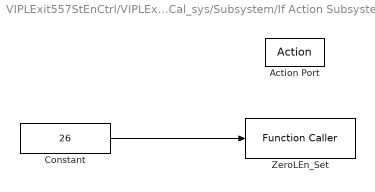
== system VIPLExit557StEnCtrl/VIPLExit557StEnCtrl_Cal_sys/Subsystem/If Action Subsystem13 ==
  Action Port : ActionPort  ActionType=then
  Constant : Constant  Value=26  OutDataTypeStr=uint8
  ZeroLEn_Set : FunctionCaller  FunctionPrototype=ZeroLEn_Set(data)  InputArgumentSpecifications=uint8(1)
  wires:
  Constant/1 -> ZeroLEn_Set/1

== system VIPLExit557StEnCtrl/VIPLExit557StEnCtrl_Cal_sys/Subsystem/If Action Subsystem14 ==
  Action Port : ActionPort  ActionType=then
  Constant : Constant  Value=26  OutDataTypeStr=uint8
  SecRwLtStBkReclnEn_Set : FunctionCaller  FunctionPrototype=SecRwLtStBkReclnEn_Set(data)  InputArgumentSpecifications=uint8(1)
  wires:
  Constant/1 -> SecRwLtStBkReclnEn_Set/1

== system VIPLExit557StEnCtrl/VIPLExit557StEnCtrl_Cal_sys/Subsystem/If Action Subsystem2 ==
  Action Port : ActionPort  ActionType=then
  Constant : Constant  Value=26  OutDataTypeStr=uint8
  SecRwLtStFwdBkwdEn_Set : FunctionCaller  FunctionPrototype=SecRwLtStFwdBkwdEn_Set(data)  InputArgumentSpecifications=uint8(1)
  wires:
  Constant/1 -> SecRwLtStFwdBkwdEn_Set/1

== system VIPLExit557StEnCtrl/VIPLExit557StEnCtrl_Cal_sys/Subsystem/If Action Subsystem3 ==
  Action Port : ActionPort  ActionType=else
  Constant : Constant  Value=26  OutDataTypeStr=uint8
  ThdRwLtStBkReclnEn_Clear : FunctionCaller  FunctionPrototype=ThdRwLtStBkReclnEn_Clear(data)  InputArgumentSpecifications=uint8(1)
  wires:
  Constant/1 -> ThdRwLtStBkReclnEn_Clear/1

== system VIPLExit557StEnCtrl/VIPLExit557StEnCtrl_Cal_sys/Subsystem/If Action Subsystem4 ==
  Action Port : ActionPort  ActionType=then
  Constant : Constant  Value=26  OutDataTypeStr=uint8
  ThdRwLtStBkReclnEn_Set : FunctionCaller  FunctionPrototype=ThdRwLtStBkReclnEn_Set(data)  InputArgumentSpecifications=uint8(1)
  wires:
  Constant/1 -> ThdRwLtStBkReclnEn_Set/1

== system VIPLExit557StEnCtrl/VIPLExit557StEnCtrl_Cal_sys/Subsystem/If Action Subsystem5 ==
  Action Port : ActionPort  ActionType=else
  Constant : Constant  Value=26  OutDataTypeStr=uint8
  ThdRwLtStFwdBkwdEn_Clear : FunctionCaller  FunctionPrototype=ThdRwLtStFwdBkwdEn_Clear(data)  InputArgumentSpecifications=uint8(1)
  wires:
  Constant/1 -> ThdRwLtStFwdBkwdEn_Clear/1

== system VIPLExit557StEnCtrl/VIPLExit557StEnCtrl_Cal_sys/Subsystem/If Action Subsystem6 ==
  Action Port : ActionPort  ActionType=then
  Constant : Constant  Value=26  OutDataTypeStr=uint8
  ThdRwLtStFwdBkwdEn_Set : FunctionCaller  FunctionPrototype=ThdRwLtStFwdBkwdEn_Set(data)  InputArgumentSpecifications=uint8(1)
  wires:
  Constant/1 -> ThdRwLtStFwdBkwdEn_Set/1

== system VIPLExit557StEnCtrl/VIPLExit557StEnCtrl_Cal_sys/Subsystem/If Action Subsystem7 ==
  Action Port : ActionPort  ActionType=else
  Constant : Constant  Value=26  OutDataTypeStr=uint8
  SecRwLtStLgrstUpwdDnwdEn_Clear : FunctionCaller  FunctionPrototype=SecRwLtStLgrstUpwdDnwdEn_Clear(data)  InputArgumentSpecifications=uint8(1)
  wires:
  Constant/1 -> SecRwLtStLgrstUpwdDnwdEn_Clear/1

== system VIPLExit557StEnCtrl/VIPLExit557StEnCtrl_Cal_sys/Subsystem/If Action Subsystem8 ==
  Action Port : ActionPort  ActionType=then
  Constant : Constant  Value=26  OutDataTypeStr=uint8
  SecRwLtStLgrstUpwdDnwdEn_Set : FunctionCaller  FunctionPrototype=SecRwLtStLgrstUpwdDnwdEn_Set(data)  InputArgumentSpecifications=uint8(1)
  wires:
  Constant/1 -> SecRwLtStLgrstUpwdDnwdEn_Set/1

== system VIPLExit557StEnCtrl/VIPLExit557StEnCtrl_Cal_sys/Subsystem/If Action Subsystem9 ==
  Action Port : ActionPort  ActionType=else
  Constant : Constant  Value=26  OutDataTypeStr=uint8
  SecRwLtStLgrstInwdOtwdEn_Clear : FunctionCaller  FunctionPrototype=SecRwLtStLgrstInwdOtwdEn_Clear(data)  InputArgumentSpecifications=uint8(1)
  wires:
  Constant/1 -> SecRwLtStLgrstInwdOtwdEn_Clear/1

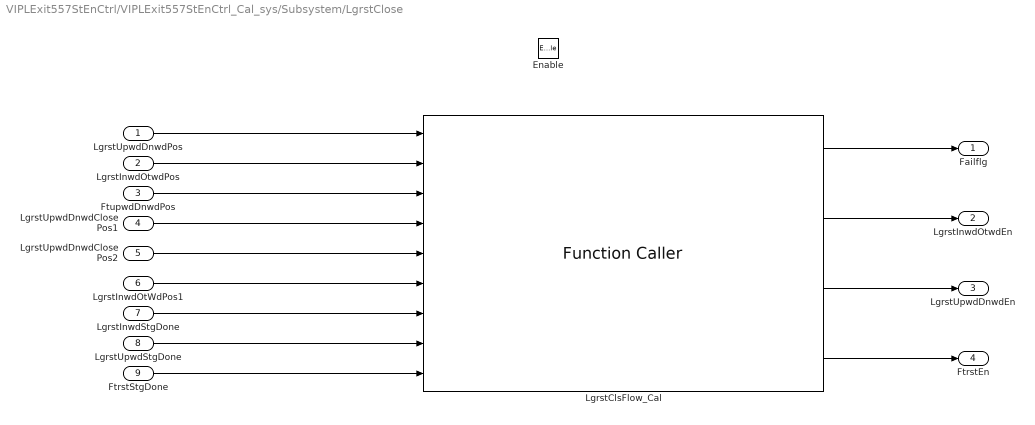
== system VIPLExit557StEnCtrl/VIPLExit557StEnCtrl_Cal_sys/Subsystem/LgrstClose ==
  LgrstUpwdDnwdPos : Inport
  LgrstInwdOtwdPos : Inport  Port=2
  FtupwdDnwdPos : Inport  Port=3
  LgrstUpwdDnwdClosePos1 : Inport  Port=4
  LgrstUpwdDnwdClosePos2 : Inport  Port=5
  LgrstInwdOtWdPos1 : Inport  Port=6
  LgrstInwdStgDone : Inport  Port=7
  LgrstUpwdStgDone : Inport  Port=8
  FtrstStgDone : Inport  Port=9
  Enable : EnablePort  StatesWhenEnabling=reset
  LgrstClsFlow_Cal : FunctionCaller  FunctionPrototype=[Failflg,LgrstInwdOtwdEn,LgrstUpwdDnwdEn,FtrstEn] = LgrstClsFlow_Cal(LgrstUpwdDnwdPos,LgrstOtwdInwdPos,FtUpwdDnwdPos,CloseDnwdPos1,CloseDnwdPos2,CloseOtwdPos1,LgrstInwdStgDone,LgrstUpwdStgDone,FtrstStgDone)  InputArgumentSpecifications=uint16(1), uint16(1), uint16(1), uint16(1), uint16(1), uint16(1), boolean(true), boolean(true), boolean(true)  OutputArgumentSpecifications=boolean(true), boolean(true), boolean(true), boolean(true)
  Failflg : Outport
  LgrstInwdOtwdEn : Outport  Port=2
  LgrstUpwdDnwdEn : Outport  Port=3
  FtrstEn : Outport  Port=4
  wires:
  LgrstClsFlow_Cal/1 -> Failflg/1
  LgrstClsFlow_Cal/4 -> FtrstEn/1
  LgrstClsFlow_Cal/3 -> LgrstUpwdDnwdEn/1
  LgrstUpwdDnwdPos/1 -> LgrstClsFlow_Cal/1
  LgrstClsFlow_Cal/2 -> LgrstInwdOtwdEn/1
  LgrstUpwdDnwdClosePos1/1 -> LgrstClsFlow_Cal/4
  LgrstUpwdStgDone/1 -> LgrstClsFlow_Cal/8
  LgrstInwdStgDone/1 -> LgrstClsFlow_Cal/7
  FtrstStgDone/1 -> LgrstClsFlow_Cal/9
  LgrstUpwdDnwdClosePos2/1 -> LgrstClsFlow_Cal/5
  LgrstInwdOtWdPos1/1 -> LgrstClsFlow_Cal/6
  LgrstInwdOtwdPos/1 -> LgrstClsFlow_Cal/2
  FtupwdDnwdPos/1 -> LgrstClsFlow_Cal/3

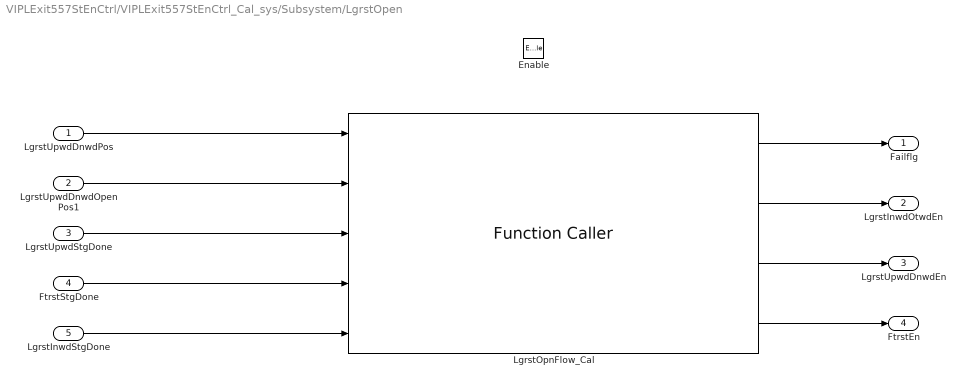
== system VIPLExit557StEnCtrl/VIPLExit557StEnCtrl_Cal_sys/Subsystem/LgrstOpen ==
  LgrstUpwdDnwdPos : Inport
  LgrstUpwdDnwdOpenPos1 : Inport  Port=2
  LgrstUpwdStgDone : Inport  Port=3
  FtrstStgDone : Inport  Port=4
  LgrstInwdStgDone : Inport  Port=5
  Enable : EnablePort  StatesWhenEnabling=reset
  LgrstOpnFlow_Cal : FunctionCaller  FunctionPrototype=[Failflg,LgrstInwdOtwdEn,LgrstUpwdDnwdEn,FtrstEn] = LgrstOpnFlow_Cal(LgrstUpwdDnwdPos,LgrstUpwdDnwdOpenPos1,LgrstUpwdStgDone,FtrstStgDone,LgrstInwdStgDone)  InputArgumentSpecifications=uint16(1), uint16(1), boolean(true), boolean(true), boolean(true)  OutputArgumentSpecifications=boolean(true), boolean(true), boolean(true), boolean(true)
  Failflg : Outport
  LgrstInwdOtwdEn : Outport  Port=2
  LgrstUpwdDnwdEn : Outport  Port=3
  FtrstEn : Outport  Port=4
  wires:
  LgrstOpnFlow_Cal/2 -> LgrstInwdOtwdEn/1
  LgrstUpwdDnwdPos/1 -> LgrstOpnFlow_Cal/1
  LgrstOpnFlow_Cal/3 -> LgrstUpwdDnwdEn/1
  FtrstStgDone/1 -> LgrstOpnFlow_Cal/4
  LgrstUpwdStgDone/1 -> LgrstOpnFlow_Cal/3
  LgrstOpnFlow_Cal/4 -> FtrstEn/1
  LgrstInwdStgDone/1 -> LgrstOpnFlow_Cal/5
  LgrstUpwdDnwdOpenPos1/1 -> LgrstOpnFlow_Cal/2
  LgrstOpnFlow_Cal/1 -> Failflg/1

== stateflow chart VIPLExit557StEnCtrl/VIPLExit557StEnCtrl_Cal_sys/Subsystem/Chart ==
  (default) -> (junction 38) : {
      | ThdRwLtStBkReclnEn = 0;
      | SecRwLtStBkReclnEn = 0;
      | SecRwLtStFrwdBkwdEn = 0;
      | SecRwLtStLgrstOtwdInwdEn = 0;
      | SecRwLtStLgrstUpwdDnwdEn = 0;
      | ThdRwLtStFwdBkwdEn = 0;
      | ZeroLEn = 0;
      | LgrstOpnEn = 0;
      | LgrstClsEn = 0;
      | }
  (junction 38) -> (junction 40) [order 1] : [IfVeSMSuSecRwLtStBkReclnUpwdDnwdPos>VIPLR2LBkReclnUpwdDnwdTrgtPos&&!SecRwLtStBkReclnStgDone]
  (junction 38) -> (junction 44) [order 2]
  (junction 40) -> (junction 42) : {SecRwLtStBkReclnEn = 1;}
  (junction 42) -> (junction 44)
  (junction 44) -> (junction 56)
  (junction 56) -> (junction 58) [order 1] : [LgrstMoveDirection == 1&& !LgrstStgDone]
  (junction 56) -> (junction 62) [order 2]
  (junction 58) -> (junction 60) : {
      | LgrstClsEn = 1;
      | }
  (junction 60) -> (junction 62)
  (junction 62) -> (junction 111)
  (junction 111) -> (junction 113) [order 1] : [IfVeSMSuSecRwLtStZeroPos >VIPLMdR2LZeroTrgtPos && !ZeroLStgDone]
  (junction 111) -> (junction 117) [order 2]
  (junction 113) -> (junction 115) : {ZeroLEn = 1;}
  (junction 115) -> (junction 117)
  (junction 117) -> (junction 147)
  (junction 147) -> (junction 149) [order 1] : [IfVeSMSuThdRwLtStBkReclnUpwdDnwdPos>VIPLR3LBkReclnUpwdDnwdTrgtPos...
      | &&!ThdRwLtStBkReclnStgDone]
  (junction 147) -> (junction 153) [order 2]
  (junction 149) -> (junction 151) : {
      | ThdRwLtStBkReclnEn = 1;
      | }
  (junction 151) -> (junction 153)
  (junction 153) -> (junction 65)
  (junction 65) -> (junction 67) [order 1] : [
      | !((IfVeSMSuSecRwLtStBkReclnUpwdDnwdPos<=VIPLR2LBkReclnUpwdDnwdTrgtPos||SecRwLtStBkReclnStgDone)&&...
      | (IfVeSMSuSecRwLtStZeroPos <=VIPLMdR2LZeroTrgtPos ||ZeroLStgDone)&&...
      | (LgrstMoveDirection !=1||LgrstStgDone)&&...
      | (R3LMdSeatOccupied||IfVeSMSuThdRwLtStBkReclnUpwdDnwdPos<=VIPLR3LBkReclnUpwdDnwdTrgtPos||ThdRwLtStBkReclnStgDone))
      | ]
  (junction 65) -> (junction 156) [order 2]
  (junction 67) -> (junction 175)
  (junction 156) -> (junction 158) [order 1] : [SecRwLtStFrwdBkwdStgDone]
  (junction 156) -> (junction 162) [order 2] : {SecRwLtStFrwdBkwdEn =1;}
  (junction 158) -> (junction 160)
  (junction 160) -> (junction 162)
  (junction 162) -> (junction 87)
  (junction 87) -> (junction 166) [order 1] : [ThdRwLtStFwdBkwdStgDone]
  (junction 87) -> (junction 170) [order 2] : {ThdRwLtStFwdBkwdEn = 1;}
  (junction 166) -> (junction 168)
  (junction 168) -> (junction 170)
  (junction 170) -> (junction 173)
  (junction 173) -> (junction 175) [order 1] : [!SecRwLtStFrwdBkwdStgDone||!ThdRwLtStFwdBkwdStgDone]
  (junction 173) -> (junction 179) [order 2]
  (junction 175) -> (junction 177)
  (junction 179) -> (junction 181) [order 1] : [ !ZeroLStgDone]
  (junction 179) -> (junction 185) [order 2]
  (junction 181) -> (junction 183) : {ZeroLEn = 1;}
  (junction 183) -> (junction 185)
  (junction 185) -> (junction 188)
  (junction 188) -> (junction 190) [order 1] : [!SecRwLtStBkReclnStgDone]
  (junction 188) -> (junction 194) [order 2]
  (junction 190) -> (junction 192) : {SecRwLtStBkReclnEn = 1;}
  (junction 192) -> (junction 194)
  (junction 194) -> (junction 197)
  (junction 197) -> (junction 199) [order 1] : [!LgrstStgDone]
  (junction 197) -> (junction 204) [order 2]
  (junction 199) -> (junction 201) : {LgrstOpnEn = 1;}
  (junction 201) -> (junction 204)
  (junction 204) -> (junction 214)
  (junction 214) -> (junction 216) [order 1] : [!ThdRwLtStBkReclnStgDone]
  (junction 214) -> (junction 220) [order 2]
  (junction 216) -> (junction 218) : {
      | ThdRwLtStBkReclnEn = 1;
      | }
  (junction 218) -> (junction 220)
  (junction 177) -> (junction 218)
  data: IfVeSMSuSecRwLtStBkReclnUpwdDnwdPos input; IfVeSMSuSecRwLtStLgrstOtwdInwdPos input; IfVeSMSuSecRwLtStLgrstUpwdDnwdPos input; SecRwLtStBkReclnStgDone input; SecRwLtStFrwdBkwdStgDone input; SecRwLtStLgrstOtwdInwdStgDone input; SecRwLtStLgrstUpwdDnwdStgDone input; ThdRwLtStBkReclnStgDone input; ThdRwLtStFwdBkwdStgDone input; VIPLR2LBkReclnUpwdDnwdTrgtPos input; VIPLR2LLgrstInwdOtwdTrgtPos input; VIPLR2LLgrstUpwdDnwdTrgtPos input; SecRwLtStBkReclnEn output boolean; SecRwLtStFrwdBkwdEn output boolean; SecRwLtStLgrstOtwdInwdEn output boolean; ThdRwLtStBkReclnEn output boolean; ThdRwLtStFwdBkwdEn output boolean; SecRwLtStLgrstUpwdDnwdEn output boolean; ZeroLStgDone input; ZeroLEn output boolean; IfVeSMSuSecRwLtStZeroPos input; VIPLMdR2LZeroTrgtPos input; VIPLR3LBkReclnUpwdDnwdTrgtPos input; R3LMdSeatOccupied input; LgrstStgDone input; IfVeSMSuThdRwLtStBkReclnUpwdDnwdPos input; LgrstMoveDirection input uint8 =0; LgrstClsEn output boolean; LgrstOpnEn output boolean
